simulink model "smlnk_hw2"  (R2019b)
settings: Solver=VariableStepAuto  StartTime=0.0  StopTime=10.0  RelTol=1e-3
undefined symbols (not defined in the file): ol, x0
settings Model: Creator=maximemeurisse  LastModifiedBy=maximemeurisse

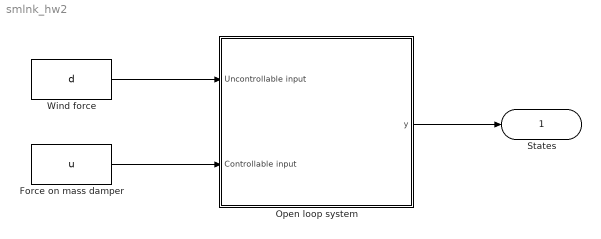
== system smlnk_hw2 ==
  Force on mass damper : FromWorkspace  VariableName=u  SampleTime=0
  Open loop system : Subsystem
  Wind force : FromWorkspace  VariableName=d  SampleTime=0
  States : Outport  SignalName=states
  wires:
  Open loop system/1(y) -> States/1
  Wind force/1 -> Open loop system/1(Uncontrollable input)
  Force on mass damper/1 -> Open loop system/2(Controllable input)

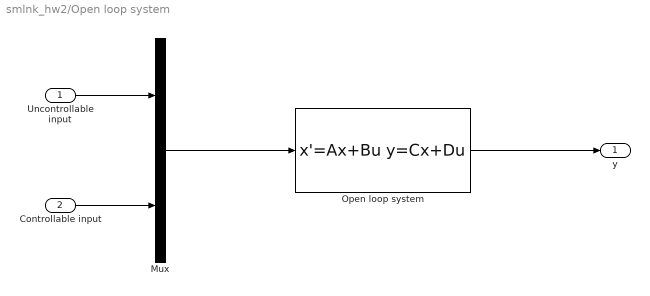
== system smlnk_hw2/Open loop system ==
  Uncontrollable input : Inport
  Controllable input : Inport  Port=2
  Mux : Mux  Inputs=2
  Open loop system : StateSpace  A=ol.A  B=ol.B  C=ol.C  D=ol.D  InitialCondition=x0
  y : Outport
  wires:
  Uncontrollable input/1 -> Mux/1
  Controllable input/1 -> Mux/2
  Open loop system/1 -> y/1
  Mux/1 -> Open loop system/1
